simulink model "EV_PMSM_ThermalModel_Revision"  (R2025b)
settings: Solver=VariableStepAuto  StartTime=0.0  StopTime=10  RelTol=1e-3
undefined symbols (not defined in the file): pmsm, Ts
libraries: fl_lib x88, nesl_utility x33, ee_lib x7, mcbcontrollergainlib x2, batteryecm_lib x1, mcbfoclib x1, mcbpositiondecoderlib x1, slpidlib x1, eePwmGeneratorTwoLevel x1
(part 2 of 2)

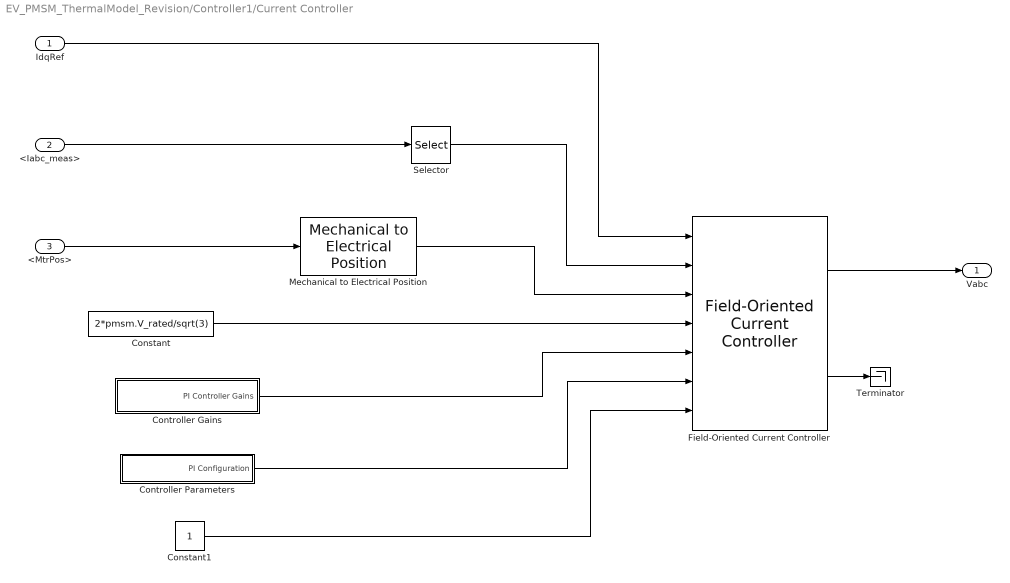
== system EV_PMSM_ThermalModel_Revision/Controller1/Current Controller ==
  IdqRef : Inport
  <Iabc_meas> : Inport  Port=2
  <MtrPos> : Inport  Port=3
  Constant : Constant  Value=2*pmsm.V_rated/sqrt(3)
  Constant1 : Constant
  Controller Gains : Subsystem
  Controller Parameters : Subsystem
  Field-Oriented Current Controller : mcbfoclib/Field-Oriented Current Controller  AngleUnit=Radians  NumberOfLUTPoints=1024  AxisAlignment=D-axis  SaturationMethod=D-Q equivalence  PWMMethod=SVM: space vector modulation
      settings: LibrarySourceBlock=mcblib/Controls/Controllers/Field-Oriented Current Controller
  Mechanical to Electrical Position : mcbpositiondecoderlib/Mechanical to Electrical Position  PolePairsInputType=Specify via dialog  NrPP=pmsm.PolePairs  selectedRange=Radians  MechOfstInputType=Specify via dialog  mechOffsetIn=0  maxAngleIn=2*pi  InputDataType=single  VariantSelect=floating-point
      settings: LibrarySourceBlock=mcblib/Sensor Decoders/Mechanical to Electrical Position
  Selector : Selector  InputPortWidth=3  IndexOptions=Index vector (dialog)  Indices=[1 2]  OutputSizes=1
  Terminator : Terminator
  Vabc : Outport
  wires:
  Field-Oriented Current Controller/1 -> Vabc/1
  <MtrPos>/1 -> Mechanical to Electrical Position/1
  IdqRef/1 -> Field-Oriented Current Controller/1
  <Iabc_meas>/1 -> Selector/1
  Controller Parameters/1(PI Configuration) -> Field-Oriented Current Controller/6
  Field-Oriented Current Controller/2 -> Terminator/1
  Constant1/1 -> Field-Oriented Current Controller/7
  Selector/1 -> Field-Oriented Current Controller/2
  Constant/1 -> Field-Oriented Current Controller/4
  Controller Gains/1(PI Controller Gains) -> Field-Oriented Current Controller/5
  Mechanical to Electrical Position/1 -> Field-Oriented Current Controller/3

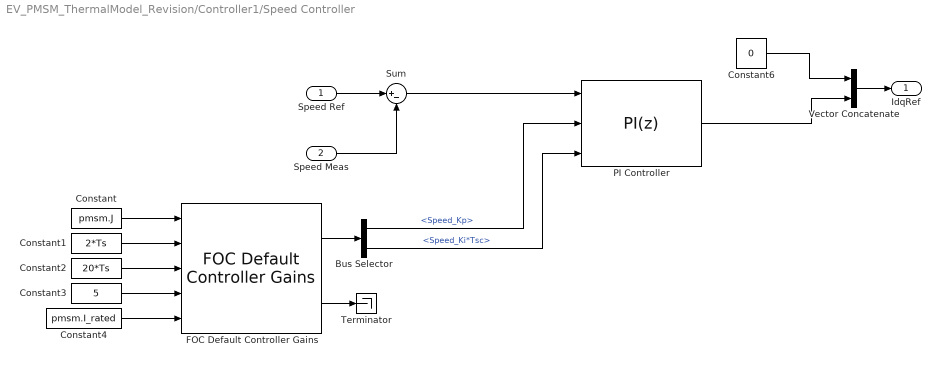
== system EV_PMSM_ThermalModel_Revision/Controller1/Speed Controller ==
  Speed Ref : Inport
  Speed Meas : Inport  Port=2
  Bus Selector : BusSelector  OutputSignals=Speed_Kp,Speed_Ki*Tsc
  Constant : Constant  Value=pmsm.J
  Constant1 : Constant  Value=2*Ts
  Constant2 : Constant  Value=20*Ts
  Constant3 : Constant  Value=5
  Constant4 : Constant  Value=pmsm.I_rated
  Constant6 : Constant  Value=0
  FOC Default Controller Gains : mcbcontrollergainlib/FOC Default Controller Gains  ControllerGainType=Empirical method  motorSelection=PMSM  unitType=SI Unit  outCurrentControlGain=off  outFWCGain=off  outSpeedControlGain=on  externalDelay=off  currentSensorDelay=50e-6  speedSensorDelay=50e-6  speedFilterDelay=0.02
      settings: LibrarySourceBlock=mcblib/Controls/Controllers/FOC Default Controller Gains
  PI Controller : slpidlib/PID Controller  Controller=PI  Form=Parallel  TimeDomain=Discrete-time  UseExternalTs=off  SampleTime=-1  IntegratorMethod=Forward Euler  FilterMethod=Forward Euler  ControllerParametersSource=external  P=1  I=1  UseKiTs=on  D=0  UseExternalDerivativeSource=off  N=100  UseFilter=on  TunerSelectOption=Transfer Function Based (PID Tuner App)  InitialConditionSource=internal  InitialConditionForIntegrator=0  InitialConditionForFilter=0  DifferentiatorICPrevScaledInput=0  ExternalReset=none  TrackingMode=off  Kt=1  LimitOutput=on  SatLimitsSource=internal  UpperSaturationLimit=pmsm.I_rated  LowerSaturationLimit=-pmsm.I_rated  LinearizeAsGain=on  AntiWindupMode=clamping  Kb=1  LimitIntegrator=on  UpperIntegratorSaturationLimit=pmsm.I_rated  LowerIntegratorSaturationLimit=-pmsm.I_rated  RndMeth=Simplest  POutMin=[]  POutMax=[]  IOutMin=[]  IOutMax=[]  DOutMin=[]  DOutMax=[]  NOutMin=[]  NOutMax=[]  SumOutMin=[]  SumOutMax=[]  SaturationOutDataTypeStr=Inherit: Inherit via back propagation  SaturationOutMin=[]  SaturationOutMax=[]  PParamMin=[]  PParamMax=[]  IParamMin=[]  IParamMax=[]  DParamMin=[]  DParamMax=[]  NParamMin=[]  NParamMax=[]  KbParamMin=[]  KbParamMax=[]  KtParamMin=[]  KtParamMax=[]  KbOutMin=[]  KbOutMax=[]  KtOutMin=[]  KtOutMax=[]  IntegratorOutMin=[]  IntegratorOutMax=[]  FilterOutMin=[]  FilterOutMax=[]  SumI1OutMin=[]  SumI1OutMax=[]  SumI2OutMin=[]  SumI2OutMax=[]  SumI3OutMin=[]  SumI3OutMax=[]  SumI4OutMin=[]  SumI4OutMax=[]  SumDOutMin=[]  SumDOutMax=[]  DifferentiatorOutMin=[]  DifferentiatorOutMax=[]  FilterDiffOutCoefMin=[]  FilterDiffOutCoefMax=[]  ReciprocalOutMin=[]  ReciprocalOutMax=[]  SumDenOutMin=[]  SumDenOutMax=[]  SumNumOutMin=[]  SumNumOutMax=[]  DivideOutMin=[]  DivideOutMax=[]  UdiffTsProdOutMin=[]  UdiffTsProdOutMax=[]  NTsProdOutMin=[]  NTsProdOutMax=[]  UintegralTsProdOutMin=[]  UintegralTsProdOutMax=[]  UngainTsProdOutMin=[]  UngainTsProdOutMax=[]  ClampingZeroOutDataTypeStr=Inherit: Inherit via back propagation  ClampingZeroOutMin=[]  ClampingZeroOutMax=[]  FilterDenConstantOutDataTypeStr=Inherit: Inherit via back propagation  FilterDenConstantOutMin=[]  FilterDenConstantOutMax=[]  PCopyOutDataTypeStr=Inherit: Inherit via back propagation  PCopyOutMin=[]  PCopyOutMax=[]  NCopyOutDataTypeStr=Inherit: Inherit via back propagation  NCopyOutMin=[]  NCopyOutMax=[]  IntegratorContinuousStateAttributes=''  IntegratorStateMustResolveToSignalObject=off  IntegratorRTWStateStorageClass=Auto  FilterContinuousStateAttributes=''  FilterStateMustResolveToSignalObject=off  FilterRTWStateStorageClass=Auto  ParallelPVariant=ExternalParameters  IdealPVariant=Disabled  IVariant=ExternalParameters  DVariant=Disabled  IntegratorVariant=Discrete  SatVariant=Enabled  AWVariant=DiscClampingParallel  PCopyVariant=Disabled  TRVariant=Disabled  FdbkBlocksVariant=Forward  IdealPFdbkVariant=Disabled  SatFdbkVariant=Disabled  DerivativeFilterVariant=Disabled  NVariant=Disabled  NCopyVariant=Disabled_SignalSpec  FilterICVariant=Disabled  IntegratorICVariant=InternalICs  ExternalResetVariant=Disabled  TRSumVariant=Passthrough  SumFdbkVariant=Disabled  SumVariant=Sum_PI  TsampFilterVariant=InternalTs  TsampNgainVariant=Passthrough  TsampIntegralVariant=Disabled_SignalSpec  ExternalSaturationOutDataTypeStr=Inherit: Same as second input  DerivativeSourceVariant=Disabled  PreIntVariant=InternalPreInt
      settings: LibrarySourceBlock=mcblib/Controls/Controllers/PI Controller
  Sum : Sum  Inputs=|+-
  Terminator : Terminator
  Vector Concatenate : Concatenate
  IdqRef : Outport
  wires:
  PI Controller/1 -> Vector Concatenate/2
  Sum/1 -> PI Controller/1
  Vector Concatenate/1 -> IdqRef/1
  Constant6/1 -> Vector Concatenate/1
  Bus Selector/2 -> PI Controller/3  "<Speed_Ki*Tsc>"
  Bus Selector/1 -> PI Controller/2  "<Speed_Kp>"
  FOC Default Controller Gains/2 -> Terminator/1
  FOC Default Controller Gains/1 -> Bus Selector/1
  Constant4/1 -> FOC Default Controller Gains/5
  Constant3/1 -> FOC Default Controller Gains/4
  Constant2/1 -> FOC Default Controller Gains/3
  Constant1/1 -> FOC Default Controller Gains/2
  Constant/1 -> FOC Default Controller Gains/1
  Speed Meas/1 -> Sum/2
  Speed Ref/1 -> Sum/1

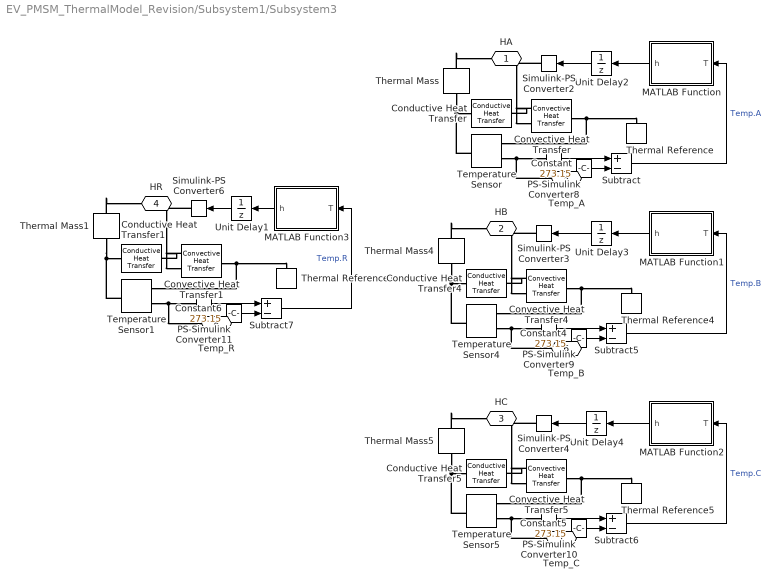
== system EV_PMSM_ThermalModel_Revision/Subsystem1/Subsystem3 ==
  Conductive Heat Transfer : fl_lib/Thermal/Thermal Elements/Conductive Heat Transfer  thermal_type=foundation.enum.ConstantVariableTabulated.Constant  wall_geometry=foundation.enum.ConductionWallGeometry.Planar  area=0.004 m^2  thickness=0.005 m  d_in=0.05 m  d_out=0.1 m  L=1 m  th_cond_min=10 W/(K*m)  th_cond=400 W/(K*m)  th_cond_TLU=[413, 401, 392, 383, 371, 357, 342] W/(K*m)  temp_TLU=[200, 273, 400, 600, 800, 1000, 1200] K  T_specify=off  T_priority=None  T=0 K  T_nominal_specify=off  T_nominal_value=1  T_nominal_unit=K  Q_specify=off  Q_priority=None  Q=0 W  Q_nominal_specify=off  Q_nominal_value=1  Q_nominal_unit=W
  Conductive Heat Transfer1 : fl_lib/Thermal/Thermal Elements/Conductive Heat Transfer  thermal_type=foundation.enum.ConstantVariableTabulated.Constant  wall_geometry=foundation.enum.ConductionWallGeometry.Planar  area=0.004 m^2  thickness=0.02 m  d_in=0.05 m  d_out=0.1 m  L=1 m  th_cond_min=10 W/(K*m)  th_cond=50 W/(K*m)  th_cond_TLU=[413, 401, 392, 383, 371, 357, 342] W/(K*m)  temp_TLU=[200, 273, 400, 600, 800, 1000, 1200] K  T_specify=off  T_priority=None  T=0 K  T_nominal_specify=off  T_nominal_value=1  T_nominal_unit=K  Q_specify=off  Q_priority=None  Q=0 W  Q_nominal_specify=off  Q_nominal_value=1  Q_nominal_unit=W
  Conductive Heat Transfer4 : fl_lib/Thermal/Thermal Elements/Conductive Heat Transfer  thermal_type=foundation.enum.ConstantVariableTabulated.Constant  wall_geometry=foundation.enum.ConductionWallGeometry.Planar  area=0.004 m^2  thickness=0.005 m  d_in=0.05 m  d_out=0.1 m  L=1 m  th_cond_min=10 W/(K*m)  th_cond=400 W/(K*m)  th_cond_TLU=[413, 401, 392, 383, 371, 357, 342] W/(K*m)  temp_TLU=[200, 273, 400, 600, 800, 1000, 1200] K  T_specify=off  T_priority=None  T=0 K  T_nominal_specify=off  T_nominal_value=1  T_nominal_unit=K  Q_specify=off  Q_priority=None  Q=0 W  Q_nominal_specify=off  Q_nominal_value=1  Q_nominal_unit=W
  Conductive Heat Transfer5 : fl_lib/Thermal/Thermal Elements/Conductive Heat Transfer  thermal_type=foundation.enum.ConstantVariableTabulated.Constant  wall_geometry=foundation.enum.ConductionWallGeometry.Planar  area=0.004 m^2  thickness=0.005 m  d_in=0.05 m  d_out=0.1 m  L=1 m  th_cond_min=10 W/(K*m)  th_cond=400 W/(K*m)  th_cond_TLU=[413, 401, 392, 383, 371, 357, 342] W/(K*m)  temp_TLU=[200, 273, 400, 600, 800, 1000, 1200] K  T_specify=off  T_priority=None  T=0 K  T_nominal_specify=off  T_nominal_value=1  T_nominal_unit=K  Q_specify=off  Q_priority=None  Q=0 W  Q_nominal_specify=off  Q_nominal_value=1  Q_nominal_unit=W
  Constant{,4..6} (4 alike) : Constant  Value=273.15
  Convective Heat Transfer{,1,4..5} (4 alike) : fl_lib/Thermal/Thermal Elements/Convective Heat Transfer  thermal_type=foundation.enum.constant_variable.variable  area=0.01 m^2  heat_tr_coeff=30 W/(K*m^2)  min_heat_tr_coeff=1e-3 W/(K*m^2)  T_specify=off  T_priority=None  T=0 K  T_nominal_specify=off  T_nominal_value=1  T_nominal_unit=K  Q_specify=off  Q_priority=None  Q=0 W  Q_nominal_specify=off  Q_nominal_value=1  Q_nominal_unit=W
      settings: InternalSimscapePortConfiguration="{\"Bottom\":[],\"Left\":[{\"id\":\"A\",\"label\":\"A\",\"type\":\"foundation.thermal.thermal\"},{\"id\":\"var_heat_tr_coeff\",\"label\":\"K\",\"type\":\"input\"}],\"Right\":[{\"id\":\"B\",\"label\":\"B\",\"type\":\"foundation.thermal.thermal\"}],\"Top\":[]}"
  MATLAB Function : MATLAB Function  TreatAsAtomicUnit=on
  MATLAB Function1 : MATLAB Function  TreatAsAtomicUnit=on
  MATLAB Function2 : MATLAB Function  TreatAsAtomicUnit=on
  MATLAB Function3 : MATLAB Function  TreatAsAtomicUnit=on
  PS-Simulink Converter{8..11} (4 alike) : nesl_utility/PS-Simulink Converter  PhysicalDomain=network_engine_domain  SubClassName=ps_output  LeftPortType=input  RightPortType=output  PseudoPeriodic=off  Frequencies=[]  VectorFormat=inherit  Unit=inherit  AffineConversion=off
  Simulink-PS Converter{2..4,6} (4 alike) : nesl_utility/Simulink-PS Converter  PhysicalDomain=network_engine_domain  SubClassName=ps_input  LeftPortType=input  RightPortType=output  PseudoPeriodic=off  Frequencies=[]  NoiseDistribution=none  NoiseParameters=[]  Unit=1  AffineConversion=off  FilteringAndDerivatives=provide  SimscapeFilterOrder=1  InputFilterTimeConstant=0.001  UdotUserProvided=0
  Subtract{,5..7} (4 alike) : Sum  Inputs=+-
  Temperature Sensor{,1,4..5} (4 alike) : fl_lib/Thermal/Thermal Sensors/Temperature Sensor  temperature_measure=foundation.enum.MeasurementReference.difference
  Thermal Mass : fl_lib/Thermal/Thermal Elements/Thermal Mass  mass_type=foundation.enum.constant_variable.constant  mass=0.5 kg  sp_heat=450 J/(K*kg)  mass_min=1e-6 kg  num_ports=foundation.enum.numPorts2.two  m_specify=off  m_priority=High  m=1 kg  m_nominal_specify=off  m_nominal_value=1  m_nominal_unit=kg  T_specify=on  T_priority=Low  T=25 degC  T_nominal_specify=off  T_nominal_value=1  T_nominal_unit=K  Q_specify=off  Q_priority=None  Q=0 W  Q_nominal_specify=off  Q_nominal_value=1  Q_nominal_unit=W
      settings: InternalSimscapePortConfiguration="{\"Bottom\":[],\"Left\":[{\"id\":\"M\",\"label\":\"\",\"type\":\"foundation.thermal.thermal\"}],\"Right\":[{\"id\":\"N\",\"label\":\"\",\"type\":\"foundation.thermal.thermal\"}],\"Top\":[]}"
  Thermal Mass1 : fl_lib/Thermal/Thermal Elements/Thermal Mass  mass_type=foundation.enum.constant_variable.constant  mass=2 kg  sp_heat=400 J/(K*kg)  mass_min=1e-6 kg  num_ports=foundation.enum.numPorts2.two  m_specify=off  m_priority=High  m=1 kg  m_nominal_specify=off  m_nominal_value=1  m_nominal_unit=kg  T_specify=on  T_priority=Low  T=25 degC  T_nominal_specify=off  T_nominal_value=1  T_nominal_unit=K  Q_specify=off  Q_priority=None  Q=0 W  Q_nominal_specify=off  Q_nominal_value=1  Q_nominal_unit=W
      settings: InternalSimscapePortConfiguration="{\"Bottom\":[],\"Left\":[{\"id\":\"M\",\"label\":\"\",\"type\":\"foundation.thermal.thermal\"}],\"Right\":[{\"id\":\"N\",\"label\":\"\",\"type\":\"foundation.thermal.thermal\"}],\"Top\":[]}"
  Thermal Mass4 : fl_lib/Thermal/Thermal Elements/Thermal Mass  mass_type=foundation.enum.constant_variable.constant  mass=0.5 kg  sp_heat=450 J/(K*kg)  mass_min=1e-6 kg  num_ports=foundation.enum.numPorts2.two  m_specify=off  m_priority=High  m=1 kg  m_nominal_specify=off  m_nominal_value=1  m_nominal_unit=kg  T_specify=on  T_priority=Low  T=25 degC  T_nominal_specify=off  T_nominal_value=1  T_nominal_unit=K  Q_specify=off  Q_priority=None  Q=0 W  Q_nominal_specify=off  Q_nominal_value=1  Q_nominal_unit=W
      settings: InternalSimscapePortConfiguration="{\"Bottom\":[],\"Left\":[{\"id\":\"M\",\"label\":\"\",\"type\":\"foundation.thermal.thermal\"}],\"Right\":[{\"id\":\"N\",\"label\":\"\",\"type\":\"foundation.thermal.thermal\"}],\"Top\":[]}"
  Thermal Mass5 : fl_lib/Thermal/Thermal Elements/Thermal Mass  mass_type=foundation.enum.constant_variable.constant  mass=0.5 kg  sp_heat=450 J/(K*kg)  mass_min=1e-6 kg  num_ports=foundation.enum.numPorts2.two  m_specify=off  m_priority=High  m=1 kg  m_nominal_specify=off  m_nominal_value=1  m_nominal_unit=kg  T_specify=on  T_priority=Low  T=25 degC  T_nominal_specify=off  T_nominal_value=1  T_nominal_unit=K  Q_specify=off  Q_priority=None  Q=0 W  Q_nominal_specify=off  Q_nominal_value=1  Q_nominal_unit=W
      settings: InternalSimscapePortConfiguration="{\"Bottom\":[],\"Left\":[{\"id\":\"M\",\"label\":\"\",\"type\":\"foundation.thermal.thermal\"}],\"Right\":[{\"id\":\"N\",\"label\":\"\",\"type\":\"foundation.thermal.thermal\"}],\"Top\":[]}"
  Thermal Reference{,1,4..5} (4 alike) : fl_lib/Thermal/Thermal Elements/Thermal Reference
  Unit Delay{1..4} (4 alike) : UnitDelay  SampleTime=-1  HasFrameUpgradeWarning=on
  HA : PMIOPort  Side=Left
  HB : PMIOPort  Port=2  Side=Left
  HC : PMIOPort  Port=3  Side=Left
  HR : PMIOPort  Port=4  Side=Right
  Temp_A : PMIOPort  Port=5  Side=Right
  Temp_B : PMIOPort  Port=6  Side=Right
  Temp_C : PMIOPort  Port=7  Side=Right
  Temp_R : PMIOPort  Port=8  Side=Right
  wires:
  Constant/1 -> Subtract/2
  MATLAB Function2/1(h) -> Unit Delay4/1
  PS-Simulink Converter10/1 -> Subtract6/1
  Unit Delay1/1 -> Simulink-PS Converter6/1
  MATLAB Function3/1(h) -> Unit Delay1/1
  Subtract6/1 -> MATLAB Function2/1(T)  "Temp.C"
  Constant5/1 -> Subtract6/2
  Subtract5/1 -> MATLAB Function1/1(T)  "Temp.B"
  MATLAB Function1/1(h) -> Unit Delay3/1
  Subtract7/1 -> MATLAB Function3/1(T)  "Temp.R"
  Subtract/1 -> MATLAB Function/1(T)  "Temp.A"
  Constant4/1 -> Subtract5/2
  Constant6/1 -> Subtract7/2
  Unit Delay3/1 -> Simulink-PS Converter3/1
  MATLAB Function/1(h) -> Unit Delay2/1
  PS-Simulink Converter11/1 -> Subtract7/1
  Unit Delay2/1 -> Simulink-PS Converter2/1
  Unit Delay4/1 -> Simulink-PS Converter4/1
  PS-Simulink Converter8/1 -> Subtract/1
  PS-Simulink Converter9/1 -> Subtract5/1
  connections:
  Convective Heat Transfer4/RConn1 -- Thermal Reference4/LConn1 -- Temperature Sensor4/RConn1
  Temperature Sensor5/RConn2 -- PS-Simulink Converter10/LConn1 -- Temp_C/RConn1
  Simulink-PS Converter6/RConn1 -- Convective Heat Transfer1/LConn2
  Temperature Sensor/RConn1 -- Thermal Reference/LConn1 -- Convective Heat Transfer/RConn1
  Temperature Sensor4/RConn2 -- PS-Simulink Converter9/LConn1 -- Temp_B/RConn1
  Thermal Mass5/LConn1 -- HC/RConn1
  Convective Heat Transfer5/RConn1 -- Thermal Reference5/LConn1 -- Temperature Sensor5/RConn1
  Temperature Sensor1/RConn2 -- PS-Simulink Converter11/LConn1 -- Temp_R/RConn1
  Temperature Sensor5/LConn1 -- Conductive Heat Transfer5/LConn1 -- Thermal Mass5/RConn1
  Temperature Sensor1/LConn1 -- Conductive Heat Transfer1/LConn1 -- Thermal Mass1/RConn1
  Simulink-PS Converter2/RConn1 -- Convective Heat Transfer/LConn2
  Temperature Sensor/LConn1 -- Conductive Heat Transfer/LConn1 -- Thermal Mass/RConn1
  Temperature Sensor4/LConn1 -- Conductive Heat Transfer4/LConn1 -- Thermal Mass4/RConn1
  Simulink-PS Converter3/RConn1 -- Convective Heat Transfer4/LConn2
  Convective Heat Transfer1/RConn1 -- Thermal Reference1/LConn1 -- Temperature Sensor1/RConn1
  Convective Heat Transfer1/LConn1 -- Conductive Heat Transfer1/RConn1
  Thermal Mass4/LConn1 -- HB/RConn1
  Convective Heat Transfer/LConn1 -- Conductive Heat Transfer/RConn1
  Temperature Sensor/RConn2 -- PS-Simulink Converter8/LConn1 -- Temp_A/RConn1
  Thermal Mass/LConn1 -- HA/RConn1
  Simulink-PS Converter4/RConn1 -- Convective Heat Transfer5/LConn2
  Convective Heat Transfer5/LConn1 -- Conductive Heat Transfer5/RConn1
  Convective Heat Transfer4/LConn1 -- Conductive Heat Transfer4/RConn1
  Thermal Mass1/LConn1 -- HR/RConn1

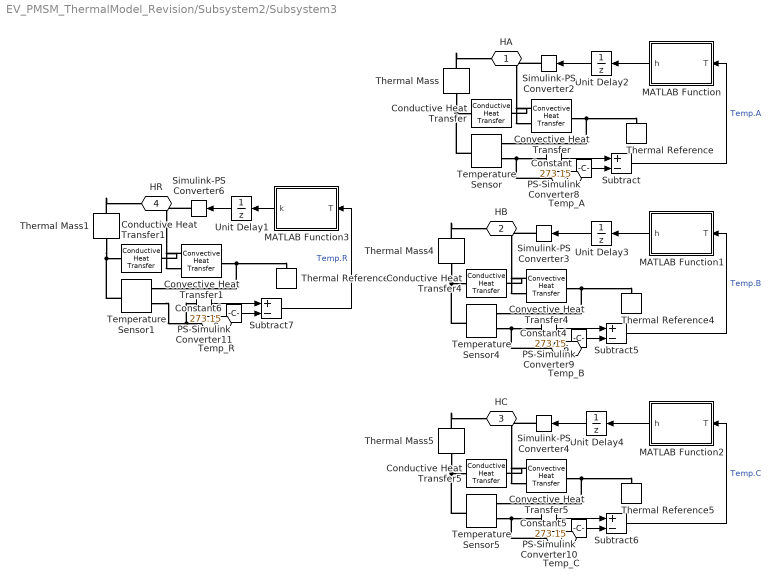
== system EV_PMSM_ThermalModel_Revision/Subsystem2/Subsystem3 ==
  Conductive Heat Transfer : fl_lib/Thermal/Thermal Elements/Conductive Heat Transfer  thermal_type=foundation.enum.ConstantVariableTabulated.Constant  wall_geometry=foundation.enum.ConductionWallGeometry.Planar  area=0.004 m^2  thickness=0.005 m  d_in=0.05 m  d_out=0.1 m  L=1 m  th_cond_min=10 W/(K*m)  th_cond=400 W/(K*m)  th_cond_TLU=[413, 401, 392, 383, 371, 357, 342] W/(K*m)  temp_TLU=[200, 273, 400, 600, 800, 1000, 1200] K  T_specify=off  T_priority=None  T=0 K  T_nominal_specify=off  T_nominal_value=1  T_nominal_unit=K  Q_specify=off  Q_priority=None  Q=0 W  Q_nominal_specify=off  Q_nominal_value=1  Q_nominal_unit=W
  Conductive Heat Transfer1 : fl_lib/Thermal/Thermal Elements/Conductive Heat Transfer  thermal_type=foundation.enum.ConstantVariableTabulated.Constant  wall_geometry=foundation.enum.ConductionWallGeometry.Planar  area=0.004 m^2  thickness=0.02 m  d_in=0.05 m  d_out=0.1 m  L=1 m  th_cond_min=10 W/(K*m)  th_cond=50 W/(K*m)  th_cond_TLU=[413, 401, 392, 383, 371, 357, 342] W/(K*m)  temp_TLU=[200, 273, 400, 600, 800, 1000, 1200] K  T_specify=off  T_priority=None  T=0 K  T_nominal_specify=off  T_nominal_value=1  T_nominal_unit=K  Q_specify=off  Q_priority=None  Q=0 W  Q_nominal_specify=off  Q_nominal_value=1  Q_nominal_unit=W
  Conductive Heat Transfer4 : fl_lib/Thermal/Thermal Elements/Conductive Heat Transfer  thermal_type=foundation.enum.ConstantVariableTabulated.Constant  wall_geometry=foundation.enum.ConductionWallGeometry.Planar  area=0.004 m^2  thickness=0.005 m  d_in=0.05 m  d_out=0.1 m  L=1 m  th_cond_min=10 W/(K*m)  th_cond=400 W/(K*m)  th_cond_TLU=[413, 401, 392, 383, 371, 357, 342] W/(K*m)  temp_TLU=[200, 273, 400, 600, 800, 1000, 1200] K  T_specify=off  T_priority=None  T=0 K  T_nominal_specify=off  T_nominal_value=1  T_nominal_unit=K  Q_specify=off  Q_priority=None  Q=0 W  Q_nominal_specify=off  Q_nominal_value=1  Q_nominal_unit=W
  Conductive Heat Transfer5 : fl_lib/Thermal/Thermal Elements/Conductive Heat Transfer  thermal_type=foundation.enum.ConstantVariableTabulated.Constant  wall_geometry=foundation.enum.ConductionWallGeometry.Planar  area=0.004 m^2  thickness=0.005 m  d_in=0.05 m  d_out=0.1 m  L=1 m  th_cond_min=10 W/(K*m)  th_cond=400 W/(K*m)  th_cond_TLU=[413, 401, 392, 383, 371, 357, 342] W/(K*m)  temp_TLU=[200, 273, 400, 600, 800, 1000, 1200] K  T_specify=off  T_priority=None  T=0 K  T_nominal_specify=off  T_nominal_value=1  T_nominal_unit=K  Q_specify=off  Q_priority=None  Q=0 W  Q_nominal_specify=off  Q_nominal_value=1  Q_nominal_unit=W
  Constant{,4..6} (4 alike) : Constant  Value=273.15
  Convective Heat Transfer{,1,4..5} (4 alike) : fl_lib/Thermal/Thermal Elements/Convective Heat Transfer  thermal_type=foundation.enum.constant_variable.variable  area=0.01 m^2  heat_tr_coeff=30 W/(K*m^2)  min_heat_tr_coeff=1e-3 W/(K*m^2)  T_specify=off  T_priority=None  T=0 K  T_nominal_specify=off  T_nominal_value=1  T_nominal_unit=K  Q_specify=off  Q_priority=None  Q=0 W  Q_nominal_specify=off  Q_nominal_value=1  Q_nominal_unit=W
      settings: InternalSimscapePortConfiguration="{\"Bottom\":[],\"Left\":[{\"id\":\"A\",\"label\":\"A\",\"type\":\"foundation.thermal.thermal\"},{\"id\":\"var_heat_tr_coeff\",\"label\":\"K\",\"type\":\"input\"}],\"Right\":[{\"id\":\"B\",\"label\":\"B\",\"type\":\"foundation.thermal.thermal\"}],\"Top\":[]}"
  MATLAB Function : MATLAB Function  TreatAsAtomicUnit=on
  MATLAB Function1 : MATLAB Function  TreatAsAtomicUnit=on
  MATLAB Function2 : MATLAB Function  TreatAsAtomicUnit=on
  MATLAB Function3 : MATLAB Function  TreatAsAtomicUnit=on
  PS-Simulink Converter{8..11} (4 alike) : nesl_utility/PS-Simulink Converter  PhysicalDomain=network_engine_domain  SubClassName=ps_output  LeftPortType=input  RightPortType=output  PseudoPeriodic=off  Frequencies=[]  VectorFormat=inherit  Unit=inherit  AffineConversion=off
  Simulink-PS Converter{2..4,6} (4 alike) : nesl_utility/Simulink-PS Converter  PhysicalDomain=network_engine_domain  SubClassName=ps_input  LeftPortType=input  RightPortType=output  PseudoPeriodic=off  Frequencies=[]  NoiseDistribution=none  NoiseParameters=[]  Unit=1  AffineConversion=off  FilteringAndDerivatives=provide  SimscapeFilterOrder=1  InputFilterTimeConstant=0.001  UdotUserProvided=0
  Subtract{,5..7} (4 alike) : Sum  Inputs=+-
  Temperature Sensor{,1,4..5} (4 alike) : fl_lib/Thermal/Thermal Sensors/Temperature Sensor  temperature_measure=foundation.enum.MeasurementReference.difference
  Thermal Mass : fl_lib/Thermal/Thermal Elements/Thermal Mass  mass_type=foundation.enum.constant_variable.constant  mass=0.5 kg  sp_heat=450 J/(K*kg)  mass_min=1e-6 kg  num_ports=foundation.enum.numPorts2.two  m_specify=off  m_priority=High  m=1 kg  m_nominal_specify=off  m_nominal_value=1  m_nominal_unit=kg  T_specify=on  T_priority=Low  T=25 degC  T_nominal_specify=off  T_nominal_value=1  T_nominal_unit=K  Q_specify=off  Q_priority=None  Q=0 W  Q_nominal_specify=off  Q_nominal_value=1  Q_nominal_unit=W
      settings: InternalSimscapePortConfiguration="{\"Bottom\":[],\"Left\":[{\"id\":\"M\",\"label\":\"\",\"type\":\"foundation.thermal.thermal\"}],\"Right\":[{\"id\":\"N\",\"label\":\"\",\"type\":\"foundation.thermal.thermal\"}],\"Top\":[]}"
  Thermal Mass1 : fl_lib/Thermal/Thermal Elements/Thermal Mass  mass_type=foundation.enum.constant_variable.constant  mass=2 kg  sp_heat=400 J/(K*kg)  mass_min=1e-6 kg  num_ports=foundation.enum.numPorts2.two  m_specify=off  m_priority=High  m=1 kg  m_nominal_specify=off  m_nominal_value=1  m_nominal_unit=kg  T_specify=on  T_priority=Low  T=25 degC  T_nominal_specify=off  T_nominal_value=1  T_nominal_unit=K  Q_specify=off  Q_priority=None  Q=0 W  Q_nominal_specify=off  Q_nominal_value=1  Q_nominal_unit=W
      settings: InternalSimscapePortConfiguration="{\"Bottom\":[],\"Left\":[{\"id\":\"M\",\"label\":\"\",\"type\":\"foundation.thermal.thermal\"}],\"Right\":[{\"id\":\"N\",\"label\":\"\",\"type\":\"foundation.thermal.thermal\"}],\"Top\":[]}"
  Thermal Mass4 : fl_lib/Thermal/Thermal Elements/Thermal Mass  mass_type=foundation.enum.constant_variable.constant  mass=0.5 kg  sp_heat=450 J/(K*kg)  mass_min=1e-6 kg  num_ports=foundation.enum.numPorts2.two  m_specify=off  m_priority=High  m=1 kg  m_nominal_specify=off  m_nominal_value=1  m_nominal_unit=kg  T_specify=on  T_priority=Low  T=25 degC  T_nominal_specify=off  T_nominal_value=1  T_nominal_unit=K  Q_specify=off  Q_priority=None  Q=0 W  Q_nominal_specify=off  Q_nominal_value=1  Q_nominal_unit=W
      settings: InternalSimscapePortConfiguration="{\"Bottom\":[],\"Left\":[{\"id\":\"M\",\"label\":\"\",\"type\":\"foundation.thermal.thermal\"}],\"Right\":[{\"id\":\"N\",\"label\":\"\",\"type\":\"foundation.thermal.thermal\"}],\"Top\":[]}"
  Thermal Mass5 : fl_lib/Thermal/Thermal Elements/Thermal Mass  mass_type=foundation.enum.constant_variable.constant  mass=0.5 kg  sp_heat=450 J/(K*kg)  mass_min=1e-6 kg  num_ports=foundation.enum.numPorts2.two  m_specify=off  m_priority=High  m=1 kg  m_nominal_specify=off  m_nominal_value=1  m_nominal_unit=kg  T_specify=on  T_priority=Low  T=25 degC  T_nominal_specify=off  T_nominal_value=1  T_nominal_unit=K  Q_specify=off  Q_priority=None  Q=0 W  Q_nominal_specify=off  Q_nominal_value=1  Q_nominal_unit=W
      settings: InternalSimscapePortConfiguration="{\"Bottom\":[],\"Left\":[{\"id\":\"M\",\"label\":\"\",\"type\":\"foundation.thermal.thermal\"}],\"Right\":[{\"id\":\"N\",\"label\":\"\",\"type\":\"foundation.thermal.thermal\"}],\"Top\":[]}"
  Thermal Reference{,1,4..5} (4 alike) : fl_lib/Thermal/Thermal Elements/Thermal Reference
  Unit Delay{1..4} (4 alike) : UnitDelay  SampleTime=-1  HasFrameUpgradeWarning=on
  HA : PMIOPort  Side=Left
  HB : PMIOPort  Port=2  Side=Left
  HC : PMIOPort  Port=3  Side=Left
  HR : PMIOPort  Port=4  Side=Right
  Temp_A : PMIOPort  Port=5  Side=Right
  Temp_B : PMIOPort  Port=6  Side=Right
  Temp_C : PMIOPort  Port=7  Side=Right
  Temp_R : PMIOPort  Port=8  Side=Right
  wires:
  PS-Simulink Converter9/1 -> Subtract5/1
  PS-Simulink Converter8/1 -> Subtract/1
  Unit Delay4/1 -> Simulink-PS Converter4/1
  Unit Delay2/1 -> Simulink-PS Converter2/1
  PS-Simulink Converter11/1 -> Subtract7/1
  MATLAB Function/1(h) -> Unit Delay2/1
  Unit Delay3/1 -> Simulink-PS Converter3/1
  Constant6/1 -> Subtract7/2
  Constant4/1 -> Subtract5/2
  Subtract/1 -> MATLAB Function/1(T)  "Temp.A"
  Subtract7/1 -> MATLAB Function3/1(T)  "Temp.R"
  MATLAB Function1/1(h) -> Unit Delay3/1
  Subtract5/1 -> MATLAB Function1/1(T)  "Temp.B"
  Constant5/1 -> Subtract6/2
  Subtract6/1 -> MATLAB Function2/1(T)  "Temp.C"
  MATLAB Function3/1(k) -> Unit Delay1/1
  Unit Delay1/1 -> Simulink-PS Converter6/1
  PS-Simulink Converter10/1 -> Subtract6/1
  MATLAB Function2/1(h) -> Unit Delay4/1
  Constant/1 -> Subtract/2
  connections:
  Thermal Mass1/LConn1 -- HR/RConn1
  Convective Heat Transfer4/LConn1 -- Conductive Heat Transfer4/RConn1
  Convective Heat Transfer5/LConn1 -- Conductive Heat Transfer5/RConn1
  Simulink-PS Converter4/RConn1 -- Convective Heat Transfer5/LConn2
  Thermal Mass/LConn1 -- HA/RConn1
  Temp_A/RConn1 -- PS-Simulink Converter8/LConn1 -- Temperature Sensor/RConn2
  Convective Heat Transfer/LConn1 -- Conductive Heat Transfer/RConn1
  Thermal Mass4/LConn1 -- HB/RConn1
  Convective Heat Transfer1/LConn1 -- Conductive Heat Transfer1/RConn1
  Temperature Sensor1/RConn1 -- Thermal Reference1/LConn1 -- Convective Heat Transfer1/RConn1
  Simulink-PS Converter3/RConn1 -- Convective Heat Transfer4/LConn2
  Thermal Mass4/RConn1 -- Conductive Heat Transfer4/LConn1 -- Temperature Sensor4/LConn1
  Thermal Mass/RConn1 -- Conductive Heat Transfer/LConn1 -- Temperature Sensor/LConn1
  Simulink-PS Converter2/RConn1 -- Convective Heat Transfer/LConn2
  Thermal Mass1/RConn1 -- Conductive Heat Transfer1/LConn1 -- Temperature Sensor1/LConn1
  Thermal Mass5/RConn1 -- Conductive Heat Transfer5/LConn1 -- Temperature Sensor5/LConn1
  Temp_R/RConn1 -- PS-Simulink Converter11/LConn1 -- Temperature Sensor1/RConn2
  Temperature Sensor5/RConn1 -- Thermal Reference5/LConn1 -- Convective Heat Transfer5/RConn1
  Thermal Mass5/LConn1 -- HC/RConn1
  Temp_B/RConn1 -- PS-Simulink Converter9/LConn1 -- Temperature Sensor4/RConn2
  Convective Heat Transfer/RConn1 -- Thermal Reference/LConn1 -- Temperature Sensor/RConn1
  Simulink-PS Converter6/RConn1 -- Convective Heat Transfer1/LConn2
  Temp_C/RConn1 -- PS-Simulink Converter10/LConn1 -- Temperature Sensor5/RConn2
  Temperature Sensor4/RConn1 -- Thermal Reference4/LConn1 -- Convective Heat Transfer4/RConn1

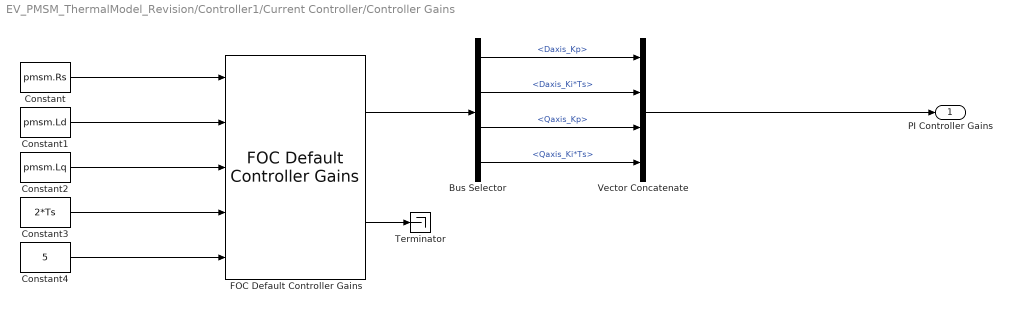
== system EV_PMSM_ThermalModel_Revision/Controller1/Current Controller/Controller Gains ==
  Bus Selector : BusSelector  OutputSignals=Daxis_Kp,Daxis_Ki*Ts,Qaxis_Kp,Qaxis_Ki*Ts
  Constant : Constant  Value=pmsm.Rs
  Constant1 : Constant  Value=pmsm.Ld
  Constant2 : Constant  Value=pmsm.Lq
  Constant3 : Constant  Value=2*Ts
  Constant4 : Constant  Value=5
  FOC Default Controller Gains : mcbcontrollergainlib/FOC Default Controller Gains  ControllerGainType=Empirical method  motorSelection=PMSM  unitType=SI Unit  outCurrentControlGain=on  outFWCGain=off  outSpeedControlGain=off  externalDelay=off  currentSensorDelay=50e-6  speedSensorDelay=50e-6  speedFilterDelay=0.02
      settings: LibrarySourceBlock=mcblib/Controls/Controllers/FOC Default Controller Gains
  Terminator : Terminator
  Vector Concatenate : Concatenate  NumInputs=4
  PI Controller Gains : Outport
  wires:
  Vector Concatenate/1 -> PI Controller Gains/1
  Bus Selector/1 -> Vector Concatenate/1  "<Daxis_Kp>"
  Bus Selector/2 -> Vector Concatenate/2  "<Daxis_Ki*Ts>"
  Bus Selector/3 -> Vector Concatenate/3  "<Qaxis_Kp>"
  Bus Selector/4 -> Vector Concatenate/4  "<Qaxis_Ki*Ts>"
  FOC Default Controller Gains/1 -> Bus Selector/1
  Constant4/1 -> FOC Default Controller Gains/5
  Constant1/1 -> FOC Default Controller Gains/2
  Constant/1 -> FOC Default Controller Gains/1
  Constant2/1 -> FOC Default Controller Gains/3
  Constant3/1 -> FOC Default Controller Gains/4
  FOC Default Controller Gains/2 -> Terminator/1

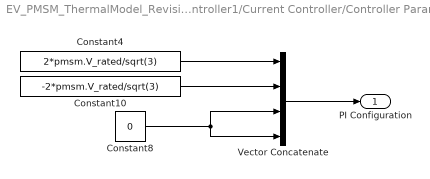
== system EV_PMSM_ThermalModel_Revision/Controller1/Current Controller/Controller Parameters ==
  Constant10 : Constant  Value=-2*pmsm.V_rated/sqrt(3)
  Constant4 : Constant  Value=2*pmsm.V_rated/sqrt(3)  OutDataTypeStr=double
  Constant8 : Constant  Value=0
  Vector Concatenate : Concatenate  NumInputs=4
  PI Configuration : Outport
  wires:
  Constant4/1 -> Vector Concatenate/1
  Constant10/1 -> Vector Concatenate/2
  Constant8/1 -> Vector Concatenate/4, Vector Concatenate/3
  Vector Concatenate/1 -> PI Configuration/1

== matlab function EV_PMSM_ThermalModel_Revision/Subsystem1/Subsystem3/MATLAB Function ==
  data: T input; h output
function h = adjust_h(T)
% T is temperature in Celsius
if T < 10
    h = 30;
elseif T < 80
    h = 15;
elseif T < 100
    h = 20;
elseif T < 120
    h = 25;
else
    h = 135;
end

== matlab function EV_PMSM_ThermalModel_Revision/Subsystem1/Subsystem3/MATLAB Function1 ==
  data: T input; h output
function h = adjust_h(T)
% T is temperature in Celsius
if T < 10
    h = 30;
elseif T < 80
    h = 15;
elseif T < 100
    h = 20;
elseif T < 120
    h = 25;
else
    h = 135;
end

== matlab function EV_PMSM_ThermalModel_Revision/Subsystem1/Subsystem3/MATLAB Function2 ==
  data: T input; h output
function h = adjust_h(T)
% T is temperature in Celsius
if T < 10
    h = 30;
elseif T < 80
    h = 15;
elseif T < 100
    h = 20;
elseif T < 120
    h = 25;
else
    h = 135;
end

== matlab function EV_PMSM_ThermalModel_Revision/Subsystem1/Subsystem3/MATLAB Function3 ==
  data: T input; h output
function h = adjust_h(T)
% T is temperature in Celsius
if T < 60
    h = 5;
elseif T < 80
    h = 10;
elseif T < 100
    h = 15;
elseif T < 120
    h = 20;
else
    h = 100;
end

== matlab function EV_PMSM_ThermalModel_Revision/Subsystem2/Subsystem3/MATLAB Function ==
  data: T input; h output
function h = adjust_h(T)
% T is temperature in Celsius
if T < 10
    h = 30;
elseif T < 80
    h = 15;
elseif T < 100
    h = 20;
elseif T < 120
    h = 25;
else
    h = 135;
end

== matlab function EV_PMSM_ThermalModel_Revision/Subsystem2/Subsystem3/MATLAB Function1 ==
  data: T input; h output
function h = adjust_h(T)
% T is temperature in Celsius
if T < 10
    h = 30;
elseif T < 80
    h = 15;
elseif T < 100
    h = 20;
elseif T < 120
    h = 25;
else
    h = 135;
end

== matlab function EV_PMSM_ThermalModel_Revision/Subsystem2/Subsystem3/MATLAB Function2 ==
  data: T input; h output
function h = adjust_h(T)
% T is temperature in Celsius
if T < 10
    h = 30;
elseif T < 80
    h = 15;
elseif T < 100
    h = 20;
elseif T < 120
    h = 25;
else
    h = 135;
end

== matlab function EV_PMSM_ThermalModel_Revision/Subsystem2/Subsystem3/MATLAB Function3 ==
  data: T input; k output
function k = adjust_k(T)
% T is temperature in Celsius
if T < 30
    k = 10;
elseif T < 40
    k= 50;
elseif T < 50
    k = 100;
elseif T < 60
    k= 150;
elseif T < 70
    k = 200;
elseif T < 80
    k= 250;
elseif T < 90
    k = 300;
elseif T < 100
    k= 350;
elseif T < 110
    k = 370;
elseif T < 120
    k = 380;
else
    k = 400;
end

== matlab function EV_PMSM_ThermalModel_Revision/Subsystem1/MATLAB Function3 ==
  data: T input; h output
function h = adjust_h(T)
% T is temperature in Celsius
if T < 60
    h = 1;
elseif T < 80
    h = 2;
elseif T < 100
    h = 3;
elseif T < 120
    h = 4;
else
    h = 5;
end
